simulink model "Control_Pc_SIM"  (R2023b)
settings: Solver=FixedStepDiscrete  StartTime=0.0  StopTime=30  FixedStep=0.01  MaxStep=0.01  RelTol=1e-3
InitFcn:
  | Ts=0.01;
StopFcn:
  | % Guardar los datos en un archivo .mat
  | guardar_datos;
  | cargar_datos;
  | % Cargar el segundo modelo
  | load('C:\Users\pablo\Desktop\control_oruga\Data\Workspace_ModeloCorrea_Cinematico.mat');
  | load_system('ModeloCorrea_Cinematico');
  | 
  | % Ejecutar el script de preparación de datos en el PreLoadFcn del segundo modelo
  | set_param('ModeloCorrea_Cinematico', 'PreLoadFcn', 'cargar_datos');
  | 
  | % Ejecutar el segundo modelo
  | set_param('ModeloCorrea_Cinematico', 'SimulationCommand', 'start');
undefined symbols (not defined in the file): DiscIntNeverNeededParam, f
libraries: simulink x3, hdlsllib x3, instrumentlib x2
settings Model: Creator=eva_g  LastModifiedBy=pablo
settings SolverCC: AlgebraicLoopSolver=TrustRegion
settings OptimizationCC: DefaultParameterBehavior=Inlined  EnhancedBackFolding=on  PassReuseOutputArgsAs=Individual arguments  ZeroExternalMemoryAtStartup=off  ZeroInternalMemoryAtStartup=off  MaxStackSize=64  OptimizeBlockOrder=speed  DifferentSizesBufferReuse=on  OptimizationCustomize=off  EfficientTunableParamExpr=on
settings DebuggingCC: ParameterTunabilityLossMsg=error  UnconnectedInputMsg=warning  UnconnectedOutputMsg=warning  UnconnectedLineMsg=warning
settings HardwareCC: ProdBitPerPointer=32  ProdBitPerSizeT=32  ProdBitPerPtrDiffT=32  ProdLargestAtomicInteger=Long  ProdLargestAtomicFloat=Double  ProdWordSize=32  ProdHWDeviceType=ARM Compatible->ARM Cortex
settings ModelReferenceCC: EnableRefExpFcnMdlSchedulingChecks=on
settings SFSimCC: MATLABDynamicMemAlloc=off
settings RTWCC: Description=Embedded Coder  SystemTargetFile=ert.tlc  TemplateMakefile=ert_default_tmf  Toolchain=Arduino ARM  BuildConfiguration=Faster Runs  DLArmComputeVersion=19.05
settings CodeAppCC: ForceParamTrailComments=on  IgnoreCustomStorageClasses=off  OperatorAnnotations=on  SimulinkDataObjDesc=on  SFDataObjDesc=on  InsertBlockDesc=on
settings ERTTargetCC: SupportContinuousTime=on  ExtModeTransport=3  ExtModeStaticAlloc=on  ExtModeStaticAllocSize=8192  ExtModeMexFile=ext_xcp  ExtModeIntrfLevel=Level2 - Open  ERTCustomFileTemplate=example_file_process.tlc

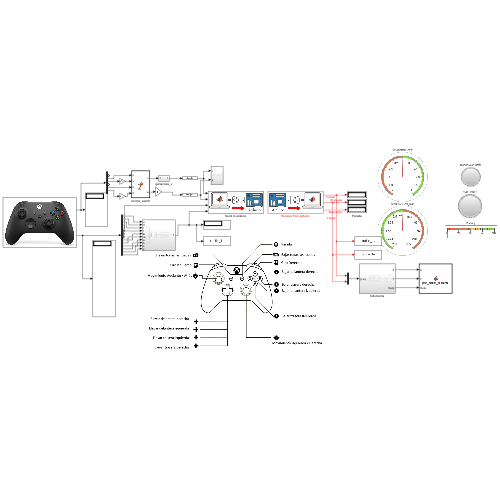
[thumbnail: Simulink's stored preview of the top-level diagram]
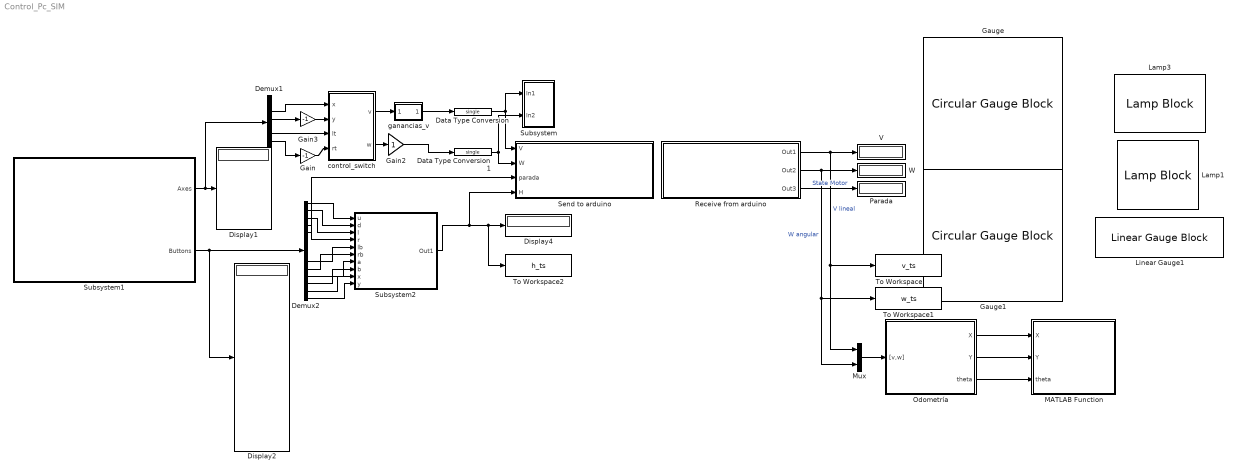
== system Control_Pc_SIM ==
  Data Type Conversion : DataTypeConversion  OutDataTypeStr=single  SaturateOnIntegerOverflow=off  RndMeth=Floor
  Data Type Conversion1 : DataTypeConversion  OutDataTypeStr=single  SaturateOnIntegerOverflow=off  RndMeth=Floor
  Demux1 : Demux  Outputs=6
  Demux2 : Demux  Outputs=14
  Display1 : Display
  Display2 : Display
  Display4 : Display
      settings: Format=binary (Stored Integer)
  Gain : Gain  Gain=-1
  Gain2 : Gain
  Gain3 : Gain  Gain=-1
  Gauge : CircularGaugeBlock  ScaleMin=-1  ScaleMax=1
  Gauge1 : CircularGaugeBlock  ScaleMin=-2.56  ScaleMax=2.56  ScaleDirection=Counterclockwise
  Lamp1 : LampBlock
  Lamp3 : LampBlock
  Linear Gauge1 : LinearGaugeBlock  TickInterval=25
  MATLAB Function : MATLAB Function  TreatAsAtomicUnit=on
  Mux : Mux  Inputs=2
  Odometría : Subsystem
  Parada : Display
  Receive from arduino : Subsystem
      mask Display: image('am.jpg'); % Use "Edit Image" on toolstrip to change.
  Send to arduino : Subsystem
      mask Display: image('ma.jpg'); % Use "Edit Image" on toolstrip to change.
  Subsystem : Subsystem
  Subsystem1 : Subsystem
      mask Display: image('mando.PNG'); % Use "Edit Image" on toolstrip to change.
  Subsystem2 : Subsystem
  To Workspace : ToWorkspace  VariableName=v_ts  SaveFormat=Timeseries  SampleTime=0.1
  To Workspace1 : ToWorkspace  VariableName=w_ts  SaveFormat=Timeseries  SampleTime=0.1
  To Workspace2 : ToWorkspace  VariableName=h_ts  SaveFormat=Timeseries  SampleTime=0.1
  V : Display
  W : Display
  control_switch : MATLAB Function  TreatAsAtomicUnit=on
  ganancias_v : Subsystem
  wires:
  Demux1/2 -> control_switch/1(x)
  Gain3/1 -> control_switch/2(y)
  control_switch/2(w) -> Gain2/1
  Gain/1 -> control_switch/4(rt)
  Receive from arduino/3(Out3) -> Parada/1  "State Motor"
  Demux2/5 -> Send to arduino/3(parada)
  Demux1/3 -> Gain3/1
  Receive from arduino/2(Out2) -> W/1, To Workspace1/1, Mux/2  "W angular"
  Gain2/1 -> Data Type Conversion1/1
  Demux1/6 -> Gain/1
  Demux1/5 -> control_switch/3(lt)
  Receive from arduino/1(Out1) -> Mux/1, To Workspace/1, V/1  "V lineal"
  Data Type Conversion/1 -> Send to arduino/1(V), Subsystem/1(In1)
  Data Type Conversion1/1 -> Send to arduino/2(W), Subsystem/2(In2)
  Subsystem1/2(Buttons) -> Display2/1, Demux2/1
  Subsystem1/1(Axes) -> Demux1/1, Display1/1
  Mux/1 -> Odometría/1("[v,w]")
  Odometría/3(theta) -> MATLAB Function/3(theta)
  Odometría/2(Y) -> MATLAB Function/2(Y)
  Odometría/1(X) -> MATLAB Function/1(X)
  control_switch/1(v) -> ganancias_v/1(In1)
  ganancias_v/1(Out1) -> Data Type Conversion/1
  Demux2/1 -> Subsystem2/1(u)
  Demux2/2 -> Subsystem2/2(d)
  Demux2/3 -> Subsystem2/3(l)
  Demux2/4 -> Subsystem2/4(r)
  Demux2/9 -> Subsystem2/5(lb)
  Demux2/10 -> Subsystem2/6(rb)
  Demux2/11 -> Subsystem2/7(a)
  Demux2/12 -> Subsystem2/8(b)
  Demux2/13 -> Subsystem2/9(x)
  Demux2/14 -> Subsystem2/10(y)
  Subsystem2/1(Out1) -> Send to arduino/4(H), To Workspace2/1, Display4/1

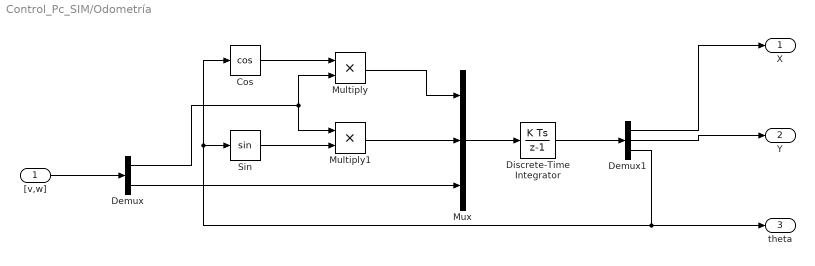
== system Control_Pc_SIM/Odometría ==
  "[v,w]" : Inport
  Cos : Trigonometry  Operator=cos
  Demux : Demux  Outputs=2
  Demux1 : Demux  Outputs=3
  Discrete-Time Integrator : DiscreteIntegrator  SampleTime=-1  ICPrevOutput=DiscIntNeverNeededParam  ICPrevScaledInput=DiscIntNeverNeededParam
  Multiply : Product
  Multiply1 : Product
  Mux : Mux  Inputs=3
  Sin : Trigonometry
  X : Outport
  Y : Outport  Port=2
  theta : Outport  Port=3
  wires:
  "[v,w]"/1 -> Demux/1
  Demux/1 -> Multiply/2, Multiply1/1
  Sin/1 -> Multiply1/2
  Cos/1 -> Multiply/1
  Multiply/1 -> Mux/1
  Multiply1/1 -> Mux/2
  Demux/2 -> Mux/3
  Mux/1 -> Discrete-Time Integrator/1
  Demux1/3 -> Sin/1, Cos/1, theta/1
  Discrete-Time Integrator/1 -> Demux1/1
  Demux1/2 -> Y/1
  Demux1/1 -> X/1

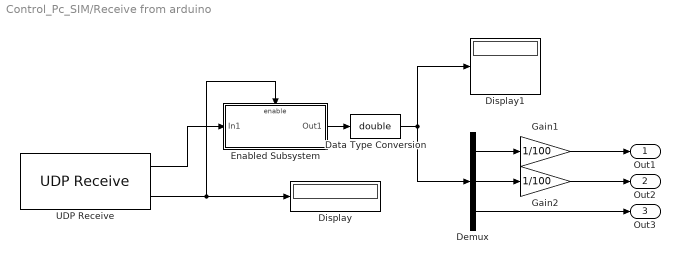
== system Control_Pc_SIM/Receive from arduino ==
  Data Type Conversion : DataTypeConversion  OutDataTypeStr=double  SaturateOnIntegerOverflow=off  RndMeth=Floor
  Demux : Demux  Outputs=3
  Display : Display
  Display1 : Display
  Enabled Subsystem : Subsystem  TreatAsAtomicUnit=on
  Gain1 : Gain  Gain=1/100
  Gain2 : Gain  Gain=1/100
  UDP Receive : instrumentlib/UDP Receive  LocalAddress=192.168.137.1  LocalPort=8888  EnablePortSharing=off  Host=192.168.137.64  Port=9090  GetLatestData=on  DataSize=[3, 1 ]  DataType=int16  ASCIIFormatting=%f,  Terminator=LF  CustomTerminator=10  ByteOrder=big-endian  EnableBlockingMode=off  Timeout=10  SampleTime=0.1  SimulateUsing=Interpreted execution
  Out1 : Outport
  Out2 : Outport  Port=2
  Out3 : Outport  Port=3
  wires:
  Demux/1 -> Gain1/1
  Gain2/1 -> Out2/1
  Demux/2 -> Gain2/1
  Demux/3 -> Out3/1
  Enabled Subsystem/1(Out1) -> Data Type Conversion/1
  UDP Receive/2 -> Display/1, Enabled Subsystem/Enable
  Gain1/1 -> Out1/1
  UDP Receive/1 -> Enabled Subsystem/1(In1)
  Data Type Conversion/1 -> Display1/1, Demux/1

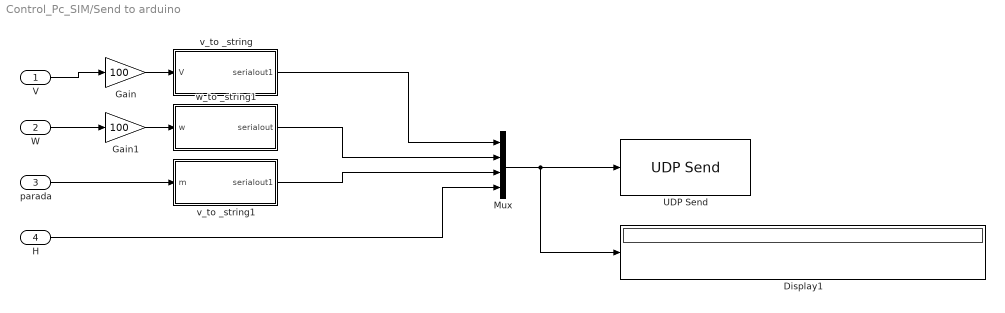
== system Control_Pc_SIM/Send to arduino ==
  V : Inport
  W : Inport  Port=2
  parada : Inport  Port=3
  H : Inport  Port=4
  Display1 : Display
  Gain : Gain  Gain=100
  Gain1 : Gain  Gain=100
  Mux : Mux
  UDP Send : instrumentlib/UDP Send  Host=192.168.137.64  Port=9090  LocalAddress=192.168.137.1  LocalPort=8888  EnablePortSharing=off  OutputDatagramPacketSize=10  ByteOrder=little-endian  EnableBlockingMode=on  SimulateUsing=Interpreted execution
  v_to _string : Subsystem
  v_to _string1 : Subsystem
  w_to _string1 : Subsystem
  wires:
  Gain/1 -> v_to _string/1(V)
  Mux/1 -> UDP Send/1, Display1/1
  W/1 -> Gain1/1
  V/1 -> Gain/1
  Gain1/1 -> w_to _string1/1(w)
  v_to _string/1(serialout1) -> Mux/1
  w_to _string1/1(serialout) -> Mux/2
  v_to _string1/1(serialout1) -> Mux/3
  parada/1 -> v_to _string1/1(m)
  H/1 -> Mux/4

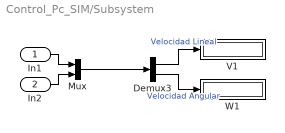
== system Control_Pc_SIM/Subsystem ==
  In1 : Inport
  In2 : Inport  Port=2
  Demux3 : Demux  Outputs=2
  Mux : Mux  Inputs=2
  V1 : Display
  W1 : Display
  wires:
  Demux3/1 -> V1/1  "Velocidad Lineal"
  Mux/1 -> Demux3/1
  In1/1 -> Mux/1
  Demux3/2 -> W1/1  "Velocidad Angular"
  In2/1 -> Mux/2

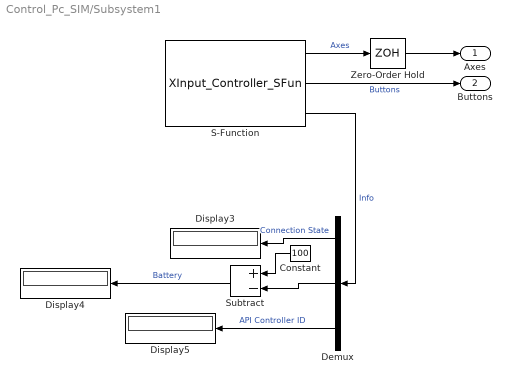
== system Control_Pc_SIM/Subsystem1 ==
  Constant : Constant  Value=100
  Demux : Demux  Outputs=3
  Display3 : Display
  Display4 : Display
  Display5 : Display
  S-Function : S-Function  FunctionName=XInput_Controller_SFun  Parameters=ControllerID  SFunctionDeploymentMode=off  EnableBusSupport=off  mask(XInput Controller){ControllerID=1}
      mask help:
      | This Block will allow you to use XInput Controllers in Simulink.
      | XInput is the most Supported API.
      | Works with XBOX 360 and XBOX ONE Controllers.
      |
      | Use 'DEMUX' to access Signals
      | Output_1 [1x6]
      |   Analog Left X, Analog Left Y,
      |   Analog Right X, Analog Right Y,
      |   Left Trigger, Right Trigger
      | Output_2 [1x14]
      |   Up, Down, Left, Right,
      |   Start, Back, Left Stick, Right Stick,
      |   Left Shoulder, Right Shoulder,
      |   A, B, X, Y
      | Output_3 [1x3]
      |   Connection State, Battery Level (1-4), Controller ID
      mask init:
      | ControllerID;   
      | blk = gcb; 
      | get_String = get_param(blk,'ControllerID');
      | ControllerID = str2double(get_String);
      mask Help:
      | Based on Microsoft XInput API
      | Therefore the maximum of conneced Gamepads per PC is 4. First Gamepad has Controller ID 1.
      | 
      | Reference:
      | https://docs.microsoft.com/en-us/windows/win32/api/_xinput/
      | 
      | Tutorial:
      | https://docs.microsoft.com/en-us/windows/win32/xinput/getting-started-with-xinput
      | 
      | Info:
      | The Analog Sticks Deadzone is coded to:
      | Deadzone = 6144;
      | 0 <= Deadzone <= 65534
      | This is smaller then Microsoft default.
      | 
      | created by Mathias Voigt
      | Technische Universität Dresden
      | 2019
      mask TypeOptions ControllerID: 1 | 2 | 3 | 4
      mask DialogControl ParameterGroupVar Prompt: Controller ID
      mask Display:
      | %% Set Block picture from user Data
      | %  (permanent, picture file not needed)
      | %  see persistent_image_allocation.m
      | 
      | %get the picture data
      | UserDataStrut = get_param(gcb, 'UserData');
      | image(UserDataStrut.Image, [0.2, 0.3, 0.6, 0.6])
      | 
      | 
      | 
      | % conventional method (does not save picture data in Simulink)
      | % image('XBOX_One_Controller_Icon.png', [0.2, 0.3, 0.6, 0.6])
      | 
      | %% Create Port Labels
      | color('blue');
      | port_label('output', 1, 'Axes');
      | port_label('output', 2, 'Buttons');
      | port_label('output', 3, 'Info');
      | 
      | 
      | %% Create S-Function Block Name
      | color('black');
      | text(0.5, 0.1, 'XInput Controller',...
      |      'horizontalAlignment', 'center',...
      |      'verticalAlignment', 'bottom');
  Subtract : Sum  Inputs=+-
  Zero-Order Hold : ZeroOrderHold  SampleTime=-1
  Axes : Outport
  Buttons : Outport  Port=2
  wires:
  Demux/1 -> Display3/1  "Connection State"
  Zero-Order Hold/1 -> Axes/1
  Demux/3 -> Display5/1  "API Controller ID"
  S-Function/1 -> Zero-Order Hold/1  "Axes"
  S-Function/3 -> Demux/1  "Info"
  S-Function/2 -> Buttons/1  "Buttons"
  Constant/1 -> Subtract/1
  Subtract/1 -> Display4/1  "Battery"
  Demux/2 -> Subtract/2

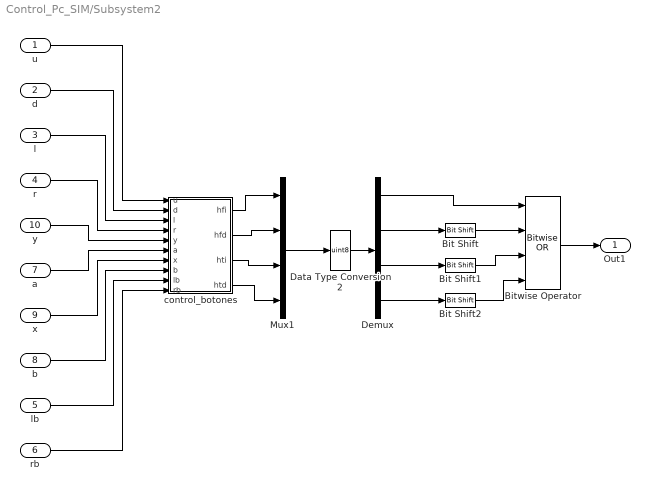
== system Control_Pc_SIM/Subsystem2 ==
  u : Inport
  d : Inport  Port=2
  l : Inport  Port=3
  r : Inport  Port=4
  lb : Inport  Port=5
  rb : Inport  Port=6
  a : Inport  Port=7
  b : Inport  Port=8
  x : Inport  Port=9
  y : Inport  Port=10
  Bit Shift : hdlsllib/Logic and Bit Operations/Bit Shift  mode=Shift Left Logical  N=1
  Bit Shift1 : hdlsllib/Logic and Bit Operations/Bit Shift  mode=Shift Left Logical  N=2
  Bit Shift2 : hdlsllib/Logic and Bit Operations/Bit Shift  mode=Shift Left Logical  N=3
  Bitwise Operator : simulink/Logic and Bit Operations/Bitwise Operator  logicop=OR  UseBitMask=off  NumInputPorts=4  BitMask=bin2dec('11011001')  BitMaskRealWorld=Stored Integer
  Data Type Conversion2 : DataTypeConversion  OutDataTypeStr=uint8  SaturateOnIntegerOverflow=off  RndMeth=Floor
  Demux : Demux
  Mux1 : Mux
  control_botones : MATLAB Function  TreatAsAtomicUnit=on
  Out1 : Outport
  wires:
  u/1 -> control_botones/1(u)
  d/1 -> control_botones/2(d)
  a/1 -> control_botones/6(a)
  l/1 -> control_botones/3(l)
  Demux/4 -> Bit Shift2/1
  r/1 -> control_botones/4(r)
  y/1 -> control_botones/5(y)
  x/1 -> control_botones/7(x)
  Bit Shift2/1 -> Bitwise Operator/4
  b/1 -> control_botones/8(b)
  lb/1 -> control_botones/9(lb)
  Demux/3 -> Bit Shift1/1
  rb/1 -> control_botones/10(rb)
  control_botones/1(hfi) -> Mux1/1
  control_botones/2(hfd) -> Mux1/2
  control_botones/3(hti) -> Mux1/3
  control_botones/4(htd) -> Mux1/4
  Mux1/1 -> Data Type Conversion2/1
  Data Type Conversion2/1 -> Demux/1
  Demux/1 -> Bitwise Operator/1
  Demux/2 -> Bit Shift/1
  Bit Shift/1 -> Bitwise Operator/2
  Bit Shift1/1 -> Bitwise Operator/3
  Bitwise Operator/1 -> Out1/1

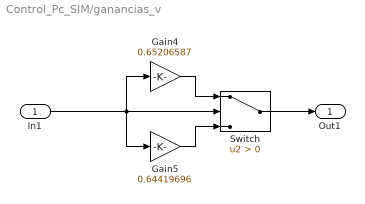
== system Control_Pc_SIM/ganancias_v ==
  In1 : Inport
  Gain4 : Gain  Gain=0.65206587
  Gain5 : Gain  Gain=0.64419696
  Switch : Switch  Criteria=u2 > Threshold  SaturateOnIntegerOverflow=off  InputSameDT=off
  Out1 : Outport
  wires:
  Switch/1 -> Out1/1
  Gain4/1 -> Switch/1
  Gain5/1 -> Switch/3
  In1/1 -> Gain4/1, Gain5/1, Switch/2

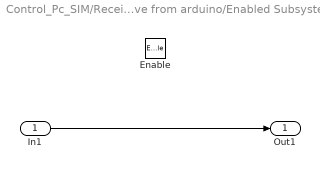
== system Control_Pc_SIM/Receive from arduino/Enabled Subsystem ==
  In1 : Inport
  Enable : EnablePort
  Out1 : Outport
  wires:
  In1/1 -> Out1/1

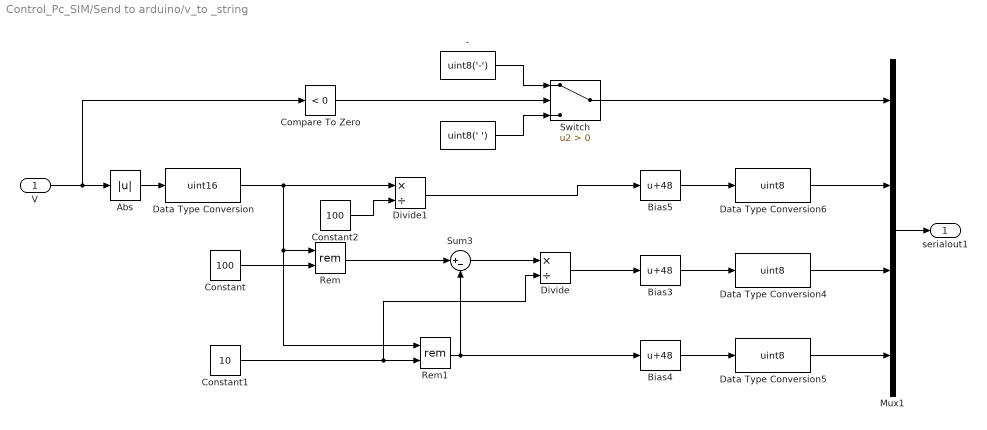
== system Control_Pc_SIM/Send to arduino/v_to _string ==
  V : Inport
  "     " : Constant  Value=uint8(' ')
  "  -" : Constant  Value=uint8('-')
  Abs : Abs  SaturateOnIntegerOverflow=off
  Bias3 : Bias  Bias=48  SaturateOnIntegerOverflow=off
  Bias4 : Bias  Bias=48  SaturateOnIntegerOverflow=off
  Bias5 : Bias  Bias=48  SaturateOnIntegerOverflow=off
  Compare To Zero : simulink/Logic and Bit Operations/Compare To Zero  relop=<  OutDataTypeStr=boolean
  Constant : Constant  Value=100  OutDataTypeStr=uint16
  Constant1 : Constant  Value=10  OutDataTypeStr=uint16
  Constant2 : Constant  Value=100  OutDataTypeStr=uint16
  Data Type Conversion : DataTypeConversion  OutDataTypeStr=uint16  SaturateOnIntegerOverflow=off  RndMeth=Floor
  Data Type Conversion4 : DataTypeConversion  OutDataTypeStr=uint8  SaturateOnIntegerOverflow=off  RndMeth=Floor
  Data Type Conversion5 : DataTypeConversion  OutDataTypeStr=uint8  SaturateOnIntegerOverflow=off  RndMeth=Floor
  Data Type Conversion6 : DataTypeConversion  OutDataTypeStr=uint8  SaturateOnIntegerOverflow=off  RndMeth=Floor
  Divide : Product  Inputs=*/
  Divide1 : Product  Inputs=*/
  Mux1 : Mux
  Rem : Math  Operator=rem
  Rem1 : Math  Operator=rem
  Sum3 : Sum  Inputs=|+-
  Switch : Switch  Criteria=u2 > Threshold  SaturateOnIntegerOverflow=off  InputSameDT=off
  serialout1 : Outport
  wires:
  Divide1/1 -> Bias5/1
  V/1 -> Compare To Zero/1, Abs/1
  Bias5/1 -> Data Type Conversion6/1
  Bias4/1 -> Data Type Conversion5/1
  Bias3/1 -> Data Type Conversion4/1
  Mux1/1 -> serialout1/1
  Data Type Conversion5/1 -> Mux1/4
  Data Type Conversion4/1 -> Mux1/3
  Data Type Conversion6/1 -> Mux1/2
  Compare To Zero/1 -> Switch/2
  "     "/1 -> Switch/3
  "  -"/1 -> Switch/1
  Switch/1 -> Mux1/1
  Constant/1 -> Rem/2
  Sum3/1 -> Divide/1
  Rem/1 -> Sum3/1
  Constant1/1 -> Divide/2, Rem1/2
  Abs/1 -> Data Type Conversion/1
  Rem1/1 -> Bias4/1, Sum3/2
  Divide/1 -> Bias3/1
  Data Type Conversion/1 -> Divide1/1, Rem1/1, Rem/1
  Constant2/1 -> Divide1/2

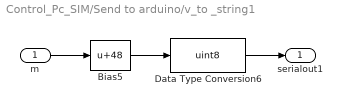
== system Control_Pc_SIM/Send to arduino/v_to _string1 ==
  m : Inport
  Bias5 : Bias  Bias=48  SaturateOnIntegerOverflow=off
  Data Type Conversion6 : DataTypeConversion  OutDataTypeStr=uint8  SaturateOnIntegerOverflow=off  RndMeth=Floor
  serialout1 : Outport
  wires:
  m/1 -> Bias5/1
  Bias5/1 -> Data Type Conversion6/1
  Data Type Conversion6/1 -> serialout1/1

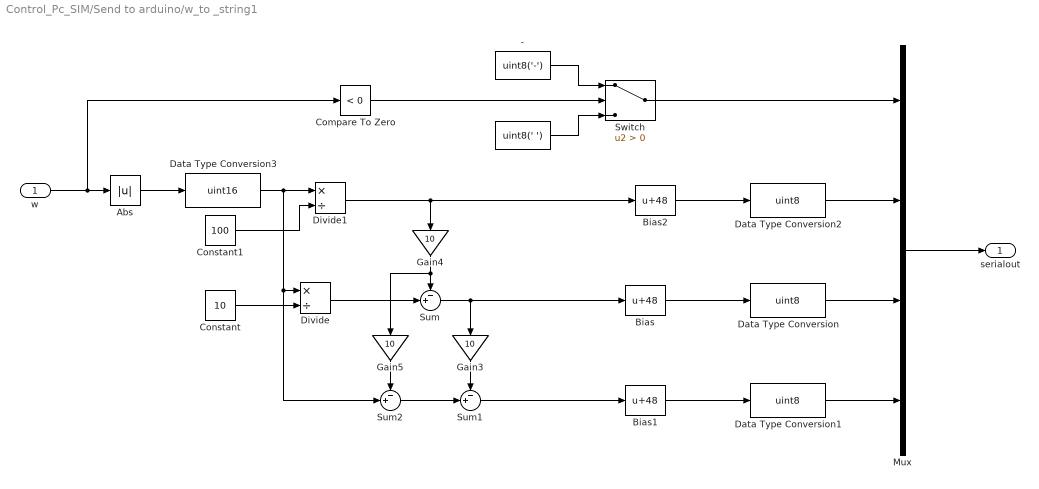
== system Control_Pc_SIM/Send to arduino/w_to _string1 ==
  w : Inport
  "     " : Constant  Value=uint8(' ')
  "  -" : Constant  Value=uint8('-')
  Abs : Abs  SaturateOnIntegerOverflow=off
  Bias : Bias  Bias=48  SaturateOnIntegerOverflow=off
  Bias1 : Bias  Bias=48  SaturateOnIntegerOverflow=off
  Bias2 : Bias  Bias=48  SaturateOnIntegerOverflow=off
  Compare To Zero : simulink/Logic and Bit Operations/Compare To Zero  relop=<  OutDataTypeStr=boolean
  Constant : Constant  Value=10  OutDataTypeStr=int16
  Constant1 : Constant  Value=100  OutDataTypeStr=int16
  Data Type Conversion : DataTypeConversion  OutDataTypeStr=uint8  SaturateOnIntegerOverflow=off  RndMeth=Floor
  Data Type Conversion1 : DataTypeConversion  OutDataTypeStr=uint8  SaturateOnIntegerOverflow=off  RndMeth=Floor
  Data Type Conversion2 : DataTypeConversion  OutDataTypeStr=uint8  SaturateOnIntegerOverflow=off  RndMeth=Floor
  Data Type Conversion3 : DataTypeConversion  OutDataTypeStr=uint16  SaturateOnIntegerOverflow=off  RndMeth=Floor
  Divide : Product  Inputs=*/
  Divide1 : Product  Inputs=*/
  Gain3 : Gain  Gain=10
  Gain4 : Gain  Gain=10
  Gain5 : Gain  Gain=10
  Mux : Mux
  Sum : Sum  Inputs=-+|
  Sum1 : Sum  Inputs=-+|
  Sum2 : Sum  Inputs=-+|
  Switch : Switch  Criteria=u2 > Threshold  SaturateOnIntegerOverflow=off  InputSameDT=off
  serialout : Outport  OutDataTypeStr=uint8
  wires:
  Sum1/1 -> Bias1/1
  Gain5/1 -> Sum2/1
  Sum2/1 -> Sum1/2
  Gain3/1 -> Sum1/1
  Gain4/1 -> Gain5/1, Sum/1
  Sum/1 -> Bias/1, Gain3/1
  Divide/1 -> Sum/2
  Data Type Conversion3/1 -> Sum2/2, Divide/1, Divide1/1
  w/1 -> Compare To Zero/1, Abs/1
  Bias2/1 -> Data Type Conversion2/1
  Divide1/1 -> Bias2/1, Gain4/1
  Bias1/1 -> Data Type Conversion1/1
  Bias/1 -> Data Type Conversion/1
  Mux/1 -> serialout/1
  Data Type Conversion1/1 -> Mux/4
  Data Type Conversion/1 -> Mux/3
  Data Type Conversion2/1 -> Mux/2
  Compare To Zero/1 -> Switch/2
  "     "/1 -> Switch/3
  "  -"/1 -> Switch/1
  Switch/1 -> Mux/1
  Abs/1 -> Data Type Conversion3/1
  Constant/1 -> Divide/2
  Constant1/1 -> Divide1/2

== matlab function Control_Pc_SIM/Subsystem2/control_botones ==
  data: u input; d input; l input; r input; y input; a input; x input; hfi output; hfd output; b input; lb input; rb input; hti output; htd output
function [hfi,hfd,hti,htd]=fcn(u,d,l,r,y,a,x,b,lb,rb)
sub=l+u+d+r; %Una suma de todos los botones de subida es equivalente a un OR
baj=a+b+x+y; %Una suma de todos los botones de bajada es equivalente a un OR
    if ((lb ==0 && rb ==0 && baj ==0) && (sub>=0))
        hfi=l; %0000 0001
        hfd=u;
        hti=d;
        htd=r;
    elseif ((lb ==0 && rb==0 && sub ==0) && (baj>=0))
        hfi=16*x; %0001 0000
        hfd=16*y;
        hti=16*a;
        htd=16*b;
    elseif ((lb>=0) && (rb==0) && (baj==0))
        hfi=lb;
        hfd=lb;
        hti=lb;
        htd=lb;        
    elseif ((rb>=0) && (lb==0) && (sub==0))
        hfi=16*rb;
        hfd=16*rb;
        hti=16*rb;
        htd=16*rb;
    else
        hfi=0;
        hfd=0;
        hti=0;
        htd=0;
    end;

== matlab function Control_Pc_SIM/control_switch ==
  data: x input; v output; y input; lt input; rt input; w output
function [v,w]=fcn(x,y,lt,rt)

    if (rt==0) && (lt==0) && ((x>=0.3) || (x<=-0.3))
        v=x;
        w=y;
    elseif (x~=0) && ((rt~=0) || (lt~=0))
        w=0;
        v=0;
    elseif (x==0) && (y==0) && (rt==0) && (lt~=0)
        w=lt;
        v=0;
    elseif (x==0) && (y==0) && (lt==0) && (rt~=0)
        w=rt;
        v=0;
    elseif (lt~=0) && (rt~=0)
        w=0;
        v=0;
    elseif (x==0) || (y==0) || (lt==0) 
        w=lt;
        v=0;
    else
        w=0;
        v=0;
    end;

== matlab function Control_Pc_SIM/MATLAB Function ==
  data: X input; Y input; theta input
function plot_robot_realtime(X, Y, theta)
    % Representación 2D del robot
    % Entradas: X, Y, theta
    
    % Dimensiones del robot
    robot_length = 1;  % Longitud del robot
    robot_width = 0.5; % Ancho del robot
    wheel_offset = 0.1;
    wheel_length = 0.2;
    wheel_width = 0.05;

    % Crear la figura
    fig = findobj('Type', 'figure', 'Name', 'Robot Simulation');
    if isempty(fig)
        fig = figure('Name', 'Robot Simulation');
        hold on;
        axis equal;
        grid on;
        xlabel('X');
        ylabel('Y');
        title('Representación 2D del Robot');
        % Configurar los límites del gráfico
        axis([-10 10 -10 10]);
    else
        figure(fig);
        clf; % Limpiar la figura antes de redibujar
        hold on;
        axis equal;
        grid on;
        xlabel('X');
        ylabel('Y');
        title('Representación 2D del Robot');
        % Configurar los límites del gráfico
        axis([-10 10 -10 10]);
    end

    % Coordenadas de las esquinas del robot antes de la rotación
    corners = [
        -robot_length/2, -robot_width/2;
         robot_length/2, -robot_width/2;
         robot_length/2,  robot_width/2;
        -robot_length/2,  robot_width/2;
    ];

    % Matriz de rotación
    R = [cos(theta), -sin(theta); sin(theta), cos(theta)];

    % Rotar y trasladar las esquinas del robot
    rotated_corners = (R * corners')';
    translated_corners = rotated_corners + [X, Y];

    % Coordenadas de las ruedas
    wheel_positions = [
        -robot_length/2 - wheel_offset, -robot_width/2 - wheel_width;
         robot_length/2 + wheel_offset, -robot_width/2 - wheel_width;
         robot_length/2 + wheel_offset,  robot_width/2 + wheel_width;
        -robot_length/2 - wheel_offset,  robot_width/2 + wheel_width;
    ];

    rotated_wheels = (R * wheel_positions')';
    translated_wheels = rotated_wheels + [X, Y];

    % Dibujar el robot y las ruedas
    fill(translated_corners(:,1), translated_corners(:,2), 'r');
    rectangle('Position', [translated_wheels(1,1) - wheel_length/2, translated_wheels(1,2) - wheel_width/2, wheel_length, wheel_width], ...
              'FaceColor', 'k');
    rectangle('Position', [translated_wheels(2,1) - wheel_length/2, translated_wheels(2,2) - wheel_width/2, wheel_length, wheel_width], ...
              'FaceColor', 'k');
    rectangle('Position', [translated_wheels(3,1) - wheel_length/2, translated_wheels(3,2) - wheel_width/2, wheel_length, wheel_width], ...
              'FaceColor', 'k');
    rectangle('Position', [translated_wheels(4,1) - wheel_length/2, translated_wheels(4,2) - wheel_width/2, wheel_length, wheel_width], ...
              'FaceColor', 'k');

    % Dibujar la dirección del robot
    quiver(X, Y, cos(theta), sin(theta), 0.5, 'b', 'LineWidth', 2, 'MaxHeadSize', 2);

    % Pausar para simular tiempo real
    pause(0.1);
end
